simulink model "cycleABC3"  (R2018b)
settings: Solver=ode1  StartTime=0.0  StopTime=Inf  FixedStep=0.005  RelTol=1e-3  EnableMultiTasking=on
libraries: simulink x5
settings Model: Creator=bbarbedette  LastModifiedBy=abenterki
settings DataIOCC: LimitDataPoints=on  SaveFormat=Array  SignalLoggingSaveFormat=ModelDataLogs
settings OptimizationCC: BlockReduction=off  OptimizeBlockIOStorage=off  BufferReuse=off  GlobalBufferReuse=off  ExpressionFolding=off  ExpressionDepthLimit=2147483647  LocalBlockOutputs=off  InitFltsAndDblsToZero=on  LifeSpan=inf  OptimizeDataStoreBuffers=off  BusAssignmentInplaceUpdate=off
settings DebuggingCC: SaveWithParameterizedLinksMsg=none  UnderspecifiedInitializationDetection=Classic  MergeDetectMultiDrivingBlocksExec=none  SolverPrmCheckMsg=warning  FcnCallInpInsideContextMsg=warning  StateNameClashWarn=warning  SFUnexpectedBacktrackingDiag=warning  SFNoUnconditionalDefaultTransitionDiag=warning  SFExecutionAtInitializationDiag=none
settings HardwareCC: ProdBitPerPointer=32  ProdBitPerSizeT=32  ProdBitPerPtrDiffT=32  ProdLargestAtomicFloat=None  ProdEndianess=BigEndian  ProdWordSize=32  ProdHWDeviceType=Specified  TargetIntDivRoundTo=Zero  TargetEndianess=BigEndian
settings ModelReferenceCC: PropagateSignalLabelsOutOfModel=off
settings SFSimCC: SimUseLocalCustomCode=off
settings RTWCC: SystemTargetFile=rti1401.tlc  MakeCommand=make_rti  TemplateMakefile=rti1401.tmf  Description=dSPACE DS1401 Hardware Platform  RTWUseLocalCustomCode=off
settings CodeAppCC: StateflowObjectComments=on
settings STFCustomTargetCC: TargetFcnLib=ansi_tfl_tmw.mat  ModelReferenceCompliant=off  GeneratePreprocessorConditionals=Disable all  MatFileLogging=on  CPPClassGenCompliant=on  GRTInterface=on  SystemTargetFile=rti1401.tlc
settings GRTTargetCC: TargetFcnLib=ansi_tfl_tmw.mat  TargetLangStandard=C89/C90 (ANSI)  ModelReferenceCompliant=off  ParMdlRefBuildCompliant=off  CompOptLevelCompliant=off  ConcurrentExecutionCompliant=off  GeneratePreprocessorConditionals=Disable all  CombineOutputUpdateFcns=off  GRTInterface=on  UseToolchainInfoCompliant=off  ExtModeMexFile=noextcomm
settings ConfigComp: CovMetricSettings=dw  CovHtmlReporting=on  CovSaveCumulativeToWorkspaceVar=on  CovSaveSingleToWorkspaceVar=on  CovExternalEMLEnable=off  CovSFcnEnable=off

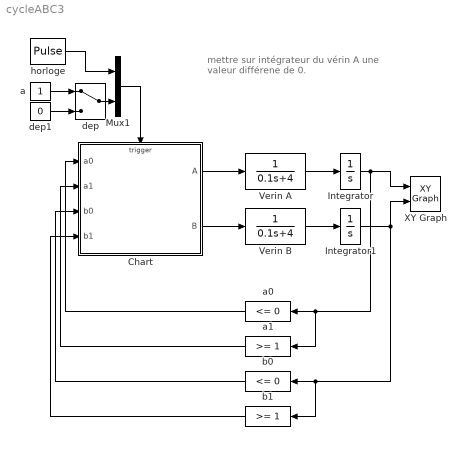
== system cycleABC3 ==
  note: mettre sur intégrateur du vérin A une
      | valeur différene de 0.
  Chart : Stateflow chart  TreatAsAtomicUnit=on
  Integrator : Integrator  InitialCondition=.5
  Integrator1 : Integrator
  Mux1 : Mux  Inputs=2
  Verin A : TransferFcn  Denominator=[0.1 4]
  Verin B : TransferFcn  Denominator=[0.1 4]
  XY Graph : simulink/Sinks/XY Graph  xmin=-3  xmax=3  ymin=-3  ymax=3  st=-1
  a : Constant
  a0 : simulink/Logic and Bit Operations/Compare To Constant  relop=<=  const=0  OutDataTypeStr=uint8  ZeroCross=off
  a1 : simulink/Logic and Bit Operations/Compare To Constant  relop=>=  const=1  OutDataTypeStr=uint8  ZeroCross=off
  b0 : simulink/Logic and Bit Operations/Compare To Constant  relop=<=  const=0  OutDataTypeStr=uint8  ZeroCross=off
  b1 : simulink/Logic and Bit Operations/Compare To Constant  relop=>=  const=1  OutDataTypeStr=uint8  ZeroCross=off
  dep : ManualSwitch
  dep1 : Constant  Value=0
  horloge : DiscretePulseGenerator  PulseType=Time based  Period=.01  PulseWidth=50
  wires:
  a/1 -> dep/1
  horloge/1 -> Mux1/1
  dep/1 -> Mux1/2
  Mux1/1 -> Chart/Trigger
  dep1/1 -> dep/2
  Chart/1(A) -> Verin A/1
  Chart/2(B) -> Verin B/1
  Verin A/1 -> Integrator/1
  Verin B/1 -> Integrator1/1
  a0/1 -> Chart/1(a0)
  a1/1 -> Chart/2(a1)
  b0/1 -> Chart/3(b0)
  b1/1 -> Chart/4(b1)
  Integrator/1 -> XY Graph/1, a0/1, a1/1
  Integrator1/1 -> XY Graph/2, b0/1, b1/1

== stateflow chart cycleABC3/Chart ==
  state X0
    en:A=0;B=0
  state X1
    en:A=1
  state X2
    en:A=0;B=1;
  state X3
    state X6 [parallel]
      settings: executionOrder=1
      state X22
        en:B=0
      (default) -> ? [order 1]
      (default) -> X22 [order 1] : [b0==1]
    state X7 [parallel]
      settings: executionOrder=2
      state X11
        en:A=-1;
      (default) -> X11
      X11 -> ? : []
  (default) -> X0
  X3 -> X0
  X0 -> X3 [order 2] : [a0==0|b0==0]
  X0 -> X1 [order 1] : dep[a0==1&b0==1]
  X1 -> X2 : [a1==1]
  X2 -> X3 : [b1==1]
  data: a0 input; a1 input; b0 input; b1 input; A output double; B output double
  events: horloge input RISING_EDGE_EVENT; dep input RISING_EDGE_EVENT
